simulink model "Prac_2_Q3_1"  (R2021a)
settings: Solver=FixedStepAuto  StartTime=0  StopTime=21600  FixedStep=300  RelTol=1e-3
values from neighbouring files (symbols this model uses):
  Cr = 100000    [Prac_2.m]
  K = 100    [Prac_2.m]
  Qf = 1000    [Prac_2.m]
  Qr1 = 1500    [Prac_2.m]
  T0 = 5    [Prac_2.m]
  Ta = 0    [Prac_2.m]
settings Model: Creator=mluser  LastModifiedBy=mluser

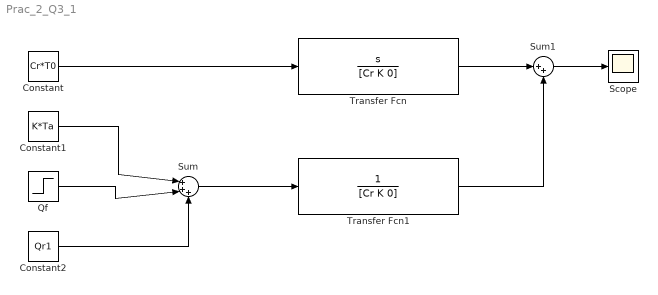
== system Prac_2_Q3_1 ==
  Constant : Constant  Value=Cr*T0
  Constant1 : Constant  Value=K*Ta
  Constant2 : Constant  Value=Qr1
  Qf : Step  Time=7200  After=Qf  SampleTime=0
  Scope : Scope
  Sum : Sum  Inputs=|+++
  Sum1 : Sum  Inputs=|++
  Transfer Fcn : TransferFcn  Numerator=[1 0]  Denominator=[Cr K 0]
  Transfer Fcn1 : TransferFcn  Denominator=[Cr K 0]
  wires:
  Constant1/1 -> Sum/1
  Qf/1 -> Sum/2
  Constant2/1 -> Sum/3
  Constant/1 -> Transfer Fcn/1
  Sum/1 -> Transfer Fcn1/1
  Transfer Fcn/1 -> Sum1/1
  Transfer Fcn1/1 -> Sum1/2
  Sum1/1 -> Scope/1
